simulink model "FD2"  (R2020b)
settings: Solver=VariableStepAuto  StartTime=0.0  StopTime=40.0  RelTol=1e-3
libraries: dspsnks4 x1, dspvision x1
settings Model: Creator=Nic  LastModifiedBy=Nic

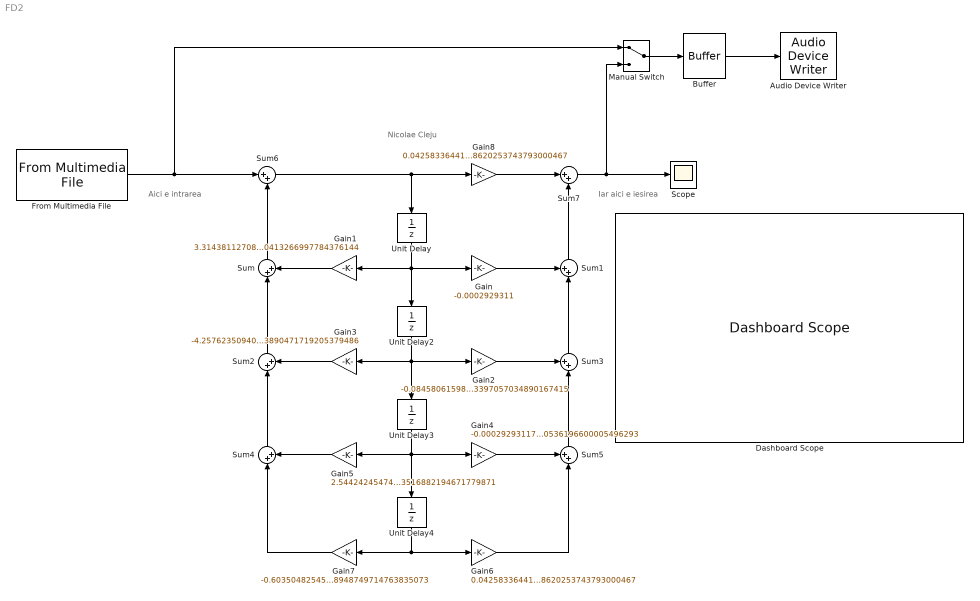
== system FD2 ==
  note: Iar aici e iesirea
  note: Aici e intrarea
  note: Nicolae Cleju
  Audio Device Writer : dspsnks4/Audio Device Writer  Driver=DirectSound  Device=Default  InheritSampleRate=on  SampleRate=44100  BitDepth=16-bit integer  BufferSize=4096  NumBuffers=10  DefaultOutputChannelMapping=on  OutputChannelMapping=1:2  OutputNumUnderrunSamples=off  DriverIdx=1  DeviceWarnFlag=''
  Buffer : Buffer  N=1024  OutputFrames=off
  Dashboard Scope : DashboardScope
  From Multimedia File : dspvision/From Multimedia File  inputFilename=D:\2020_2021\PSS\Work\L04_5407\Labs_Sample.wav  readRange=[1 Inf]  loop=on  numPlays=inf  outputStreams=Audio only  videoDataType=single  audioDataType=double  inheritSampleTime=on  userDefinedSampleTime=1/30  noAudioOutput=off  isIntensityVideo=off  fourcc=RGB  colorVideoFormat=Separate color signals  outputEOF=off  dataOrg=Column-major  audioFrameSize=1  computeAudioFrameSize=off  outSamplingMode=Sample based
  Gain : Gain  Gain=-0.0002929311
  Gain1 : Gain  Gain=3.314381127081814426560413266997784376144
  Gain2 : Gain  Gain=-0.084580615987417118173397057034890167415
  Gain3 : Gain  Gain=-4.257623509406780470953890471719205379486
  Gain4 : Gain  Gain=-0.000292931179123129270536196600005496293
  Gain5 : Gain  Gain=2.54424245474770893693516882194671779871
  Gain6 : Gain  Gain=0.042583364410483111328620253743793000467
  Gain7 : Gain  Gain=-0.603504825452040205568948749714763835073
  Gain8 : Gain  Gain=0.042583364410483111328620253743793000467
  Manual Switch : ManualSwitch
  Scope : Scope
  Sum{,2,4,6..7} (5 alike) : Sum  Inputs=|++
  Sum1 : Sum  Inputs=++|
  Sum3 : Sum  Inputs=++|
  Sum5 : Sum  Inputs=++|
  Unit Delay{,2..4} (4 alike) : UnitDelay  SampleTime=-1  HasFrameUpgradeWarning=on
  wires:
  Unit Delay/1 -> Unit Delay2/1, Gain1/1, Gain/1
  Gain1/1 -> Sum/2
  Gain/1 -> Sum1/1
  Gain2/1 -> Sum3/1
  Gain3/1 -> Sum2/2
  Unit Delay2/1 -> Unit Delay3/1, Gain3/1, Gain2/1
  Gain5/1 -> Sum4/2
  Unit Delay3/1 -> Unit Delay4/1, Gain5/1, Gain4/1
  Gain4/1 -> Sum5/1
  Gain7/1 -> Sum4/1
  Unit Delay4/1 -> Gain7/1, Gain6/1
  Gain6/1 -> Sum5/2
  Sum5/1 -> Sum3/2
  Sum3/1 -> Sum1/2
  Sum4/1 -> Sum2/1
  Sum2/1 -> Sum/1
  Sum/1 -> Sum6/2
  Sum6/1 -> Unit Delay/1, Gain8/1
  Gain8/1 -> Sum7/1
  Sum1/1 -> Sum7/2
  Sum7/1 -> Manual Switch/2, Scope/1
  From Multimedia File/1 -> Manual Switch/1, Sum6/1
  Buffer/1 -> Audio Device Writer/1
  Manual Switch/1 -> Buffer/1
